simulink model "USRP_selfCheck"  (R2020a)
settings: Solver=FixedStepAuto  StartTime=0.0  StopTime=inf  RelTol=1e-3
libraries: commsdrhw_v2 x2, dspsrcs4 x1
settings Model: SimulationMode=rapid-accelerator  Creator=longt  LastModifiedBy=longt
settings DataIOCC: SaveOutput=off  SignalLogging=off  DSMLogging=off  SaveTime=off  ReturnWorkspaceOutputs=off

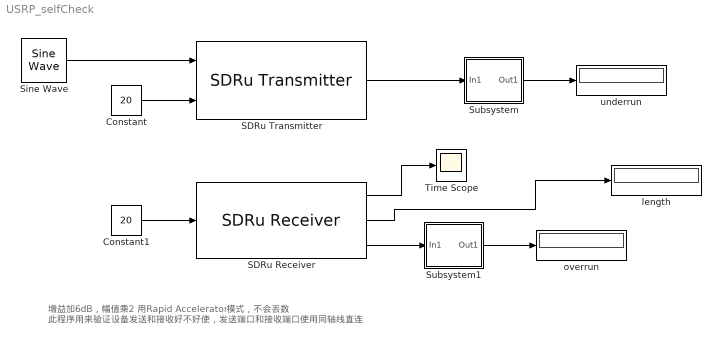
== system USRP_selfCheck ==
  note: 增益加6dB，幅值乘2
      | 用Rapid Accelerator模式，不会丢数
      | 此程序用来验证设备发送和接收好不好使，发送端口和接收端口使用同轴线直连
  Constant : Constant  Value=20
  Constant1 : Constant  Value=20
  SDRu Receiver : commsdrhw_v2/SDRu Receiver  rxtx=rx  initializeIPAddress=0  devMap=10  USRP2_IP=192.168.10.2  USRP_IP_X300=192.168.10.2  USRP_IP_X310=No devices found  USRP_IP_N300=192.168.10.2  USRP_IP_N310=192.168.10.2  USRP_IP_N320=192.168.10.2  USRP_serialNumB200=No devices found  USRP_serialNumB210=315F337  platform=B210  prevPlatform=B210  lastIPAddressPopup=192.168.10.2  USRP_ID=315F337  LastIPAddress=192.168.10.2  IsTwinRXDaughterboard=off  EnableTwinRXPhaseSync=off  losrc=0  ChannelMapping=1  centerFrequencySrc=Dialog  centerFrequency=1.57542e9  loOffsetSrc=Dialog  loOffset=0  gainSrc=Input port  gain=32  PPSSource=Internal  clockSource=Internal  masterClkRateParam=32000000  masterClkRateB200=32e6  masterClkRateB210=32e6  masterClkRateX300=200e6  masterClkRateX310=200e6  masterClkRateN300=125e6  masterClkRateN310=125e6  masterClkRateN320=200e6  masterClkRate=100e6  masterClkRateTwinRX=200e6  decimInterpSrc=Dialog  decimInterpPort=512  lastDecimSource=Dialog  decimInterp=512  USRP2_IP_NUM=[51 49 53 70 51 51 55]  sampleRate=62500  sampleTime=1.6e-05  TransportDataType=int16  overrunUnderrunPort=on  outputDatatype=Same as transport data type  frameLength=6250  HOST_DATA_PORT=0  HOST_CONTROL_PORT=0  USRP2_DATA_PORT=0  USRP2_CONTROL_PORT=0  bufferMode=Continuous streaming  EnableBurstMode=off  NumFramesInBurst=100
      settings: SourceProductBaseCode=USRP
  SDRu Transmitter : commsdrhw_v2/SDRu Transmitter  rxtx=tx  initializeIPAddress=0  devMap=0  USRP2_IP=192.168.10.2  USRP_IP_X300=192.168.10.2  USRP_IP_X310=192.168.10.2  USRP_IP_N300=No devices found  USRP_IP_N310=192.168.10.2  USRP_IP_N320=No devices found  USRP_serialNumB200=No devices found  USRP_serialNumB210=315F337  platform=B210  prevPlatform=B210  lastIPAddressPopup=192.168.10.2  USRP_ID=315F337  LastIPAddress=192.168.10.2  ChannelMapping=1  centerFrequencySrc=Dialog  centerFrequency=1.57542e9  loOffsetSrc=Dialog  loOffset=0  gainSrc=Input port  gain=8  PPSSource=Internal  clockSource=Internal  masterClkRateParam=32000000  masterClkRateB200=32e6  masterClkRateB210=32e6  masterClkRateX300=200e6  masterClkRateX310=200e6  masterClkRateN300=125e6  masterClkRateN310=125e6  masterClkRateN320=200e6  decimInterpSrc=Dialog  lastDecimSource=Dialog  decimInterp=512  USRP2_IP_NUM=[51 49 53 70 51 51 55]  frameLength=362  sampleRate=62500  TransportDataType=int16  outputDatatype=Same as transport data type  overrunUnderrunPort=on  sampleTime=5.12e-06  dboardInfo=|  HOST_DATA_PORT=30000  HOST_CONTROL_PORT=30001  USRP2_DATA_PORT=32769  USRP2_CONTROL_PORT=32768  bufferMode=Continuous streaming  EnableBurstMode=off  NumFramesInBurst=100
      | dbid: 0
      |           dbName: 'no db found'
      |          freqMin: 0
      |          freqMax: 0
      |          gainMin: 0
      |          gainMax: 0
      |     gainStepSize: 0
      settings: SourceProductBaseCode=USRP
  Sine Wave : dspsrcs4/Sine Wave  Amplitude=1  Frequency=500  Phase=0  SampleMode=Discrete  OutComplex=Complex  CompMethod=Trigonometric fcn  TableSize=Speed  SampleTime=1/62500  SamplesPerFrame=6250  ResetState=Restart at time zero  OutputFrames=off  dataType=double  wordLen=16  udDataType=sfix(16)  fracBitsMode=Best precision  numFracBits=15  OutDataTypeStr=double  LastOutDataTypeStr=double
  Subsystem : Subsystem
  Subsystem1 : Subsystem
  Time Scope : Scope
  length : Display
  overrun : Display
  underrun : Display
  wires:
  Sine Wave/1 -> SDRu Transmitter/1
  Subsystem/1(Out1) -> underrun/1
  SDRu Transmitter/1 -> Subsystem/1(In1)
  SDRu Receiver/3 -> Subsystem1/1(In1)
  Subsystem1/1(Out1) -> overrun/1
  Constant/1 -> SDRu Transmitter/2
  Constant1/1 -> SDRu Receiver/1
  SDRu Receiver/1 -> Time Scope/1
  SDRu Receiver/2 -> length/1

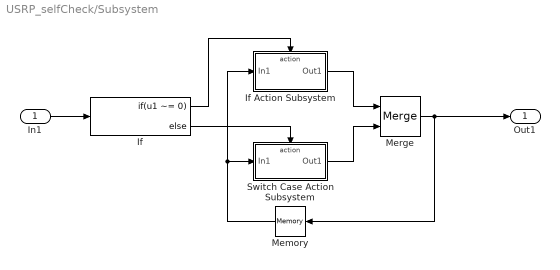
== system USRP_selfCheck/Subsystem ==
  In1 : Inport
  If : If  IfExpression=u1 ~= 0
  If Action Subsystem : Subsystem  TreatAsAtomicUnit=on
  Memory : Memory
  Merge : Merge
  Switch Case Action Subsystem : Subsystem  TreatAsAtomicUnit=on
  Out1 : Outport  VectorParamsAs1DForOutWhenUnconnected=off
  wires:
  Switch Case Action Subsystem/1(Out1) -> Merge/2
  If Action Subsystem/1(Out1) -> Merge/1
  Merge/1 -> Out1/1, Memory/1
  Memory/1 -> Switch Case Action Subsystem/1(In1), If Action Subsystem/1(In1)
  In1/1 -> If/1
  If/1 -> If Action Subsystem/Action
  If/2 -> Switch Case Action Subsystem/Action

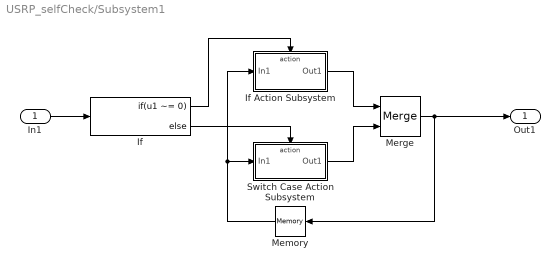
== system USRP_selfCheck/Subsystem1 ==
  In1 : Inport
  If : If  IfExpression=u1 ~= 0
  If Action Subsystem : Subsystem  TreatAsAtomicUnit=on
  Memory : Memory
  Merge : Merge
  Switch Case Action Subsystem : Subsystem  TreatAsAtomicUnit=on
  Out1 : Outport  VectorParamsAs1DForOutWhenUnconnected=off
  wires:
  If/2 -> Switch Case Action Subsystem/Action
  If/1 -> If Action Subsystem/Action
  In1/1 -> If/1
  Memory/1 -> If Action Subsystem/1(In1), Switch Case Action Subsystem/1(In1)
  Merge/1 -> Memory/1, Out1/1
  If Action Subsystem/1(Out1) -> Merge/1
  Switch Case Action Subsystem/1(Out1) -> Merge/2

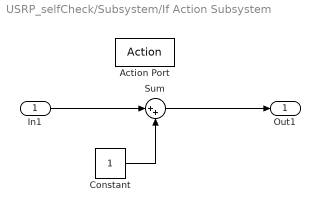
== system USRP_selfCheck/Subsystem/If Action Subsystem ==
  In1 : Inport
  Action Port : ActionPort  ActionPortLabel=if(u1 ~= 0)
  Constant : Constant
  Sum : Sum  Inputs=|++
  Out1 : Outport  VectorParamsAs1DForOutWhenUnconnected=off
  wires:
  Sum/1 -> Out1/1
  In1/1 -> Sum/1
  Constant/1 -> Sum/2

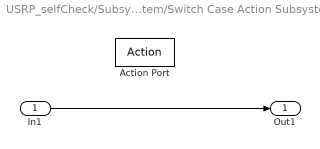
== system USRP_selfCheck/Subsystem/Switch Case Action Subsystem ==
  In1 : Inport
  Action Port : ActionPort  ActionPortLabel=else
  Out1 : Outport  VectorParamsAs1DForOutWhenUnconnected=off
  wires:
  In1/1 -> Out1/1

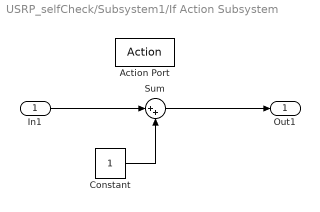
== system USRP_selfCheck/Subsystem1/If Action Subsystem ==
  In1 : Inport
  Action Port : ActionPort  ActionPortLabel=if(u1 ~= 0)
  Constant : Constant
  Sum : Sum  Inputs=|++
  Out1 : Outport  VectorParamsAs1DForOutWhenUnconnected=off
  wires:
  Constant/1 -> Sum/2
  In1/1 -> Sum/1
  Sum/1 -> Out1/1

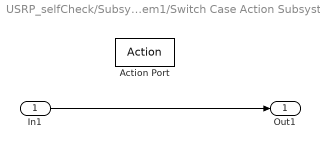
== system USRP_selfCheck/Subsystem1/Switch Case Action Subsystem ==
  In1 : Inport
  Action Port : ActionPort  ActionPortLabel=else
  Out1 : Outport  VectorParamsAs1DForOutWhenUnconnected=off
  wires:
  In1/1 -> Out1/1
